simulink model "BirdHeadModel2"  (R2023a)
settings: Solver=VariableStepAuto  StartTime=0.0  StopTime=30  RelTol=1e-3
values from neighbouring files (symbols this model uses):
  dt = 0.002    [LaunchBirdHeadModel2.m]    (also in LaunchBirdHeadModelControlled.m; LaunchBirdHeadModelControlled_MovementControl.m; PlotMovementControl.m; PlotPositionControl.m)
  g = 9.81    [LaunchBirdHeadModel2.m]    (also in LaunchBirdHeadModelControlled.m; LaunchBirdHeadModelControlled_MovementControl.m; PlotMovementControl.m; PlotPositionControl.m)
  I_by = 0.00001    (= 1e-05)    [LaunchBirdHeadModel2.m]    (also in LaunchBirdHeadModelControlled.m; LaunchBirdHeadModelControlled_MovementControl.m; PlotMovementControl.m; PlotPositionControl.m)
  I_hy = 0.00001    (= 1e-05)    [LaunchBirdHeadModel2.m]    (also in LaunchBirdHeadModelControlled.m; LaunchBirdHeadModelControlled_MovementControl.m; PlotMovementControl.m; PlotPositionControl.m)
  Kp = [20  0; 0  20]    [CondIni-1010Kp201Kv101.mat]    (also in Kp101Kv51.mat = [20  0; 0  1]; Kp11Kv051.mat = [1  0; 0  1]; Kp11Kv11.mat = [1  0; 0  1]; Kp11Kv21.mat = [1  0; 0  1])
  Kv = [10  0; 0  10]    [CondIni-1010Kp201Kv101.mat]    (also in Kp101Kv51.mat = [5  0; 0  1]; Kp11Kv051.mat = [0.5  0; 0  1]; Kp11Kv11.mat = [1  0; 0  1]; Kp11Kv21.mat = [2  0; 0  1])
  l_b = 0.05    [LaunchBirdHeadModel2.m]    (also in LaunchBirdHeadModelControlled.m; LaunchBirdHeadModelControlled_MovementControl.m; PlotMovementControl.m; PlotPositionControl.m)
  l_h = 0.04    [LaunchBirdHeadModel2.m]    (also in LaunchBirdHeadModelControlled.m; LaunchBirdHeadModelControlled_MovementControl.m; PlotMovementControl.m; PlotPositionControl.m)
  m_h = 0.005    [LaunchBirdHeadModel2.m]    (also in LaunchBirdHeadModelControlled.m; LaunchBirdHeadModelControlled_MovementControl.m; PlotMovementControl.m; PlotPositionControl.m)
settings Model: Creator=coquet  LastModifiedBy=coquet

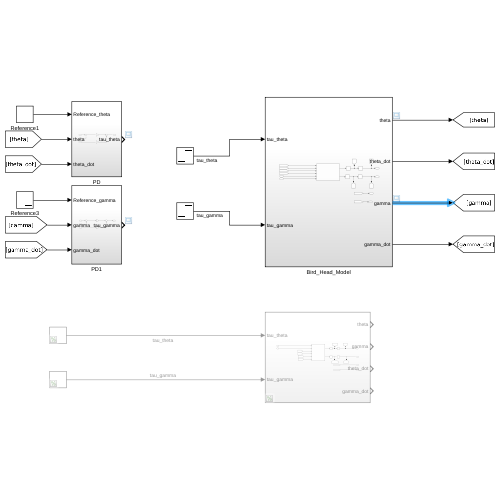
[thumbnail: Simulink's stored preview of the top-level diagram]
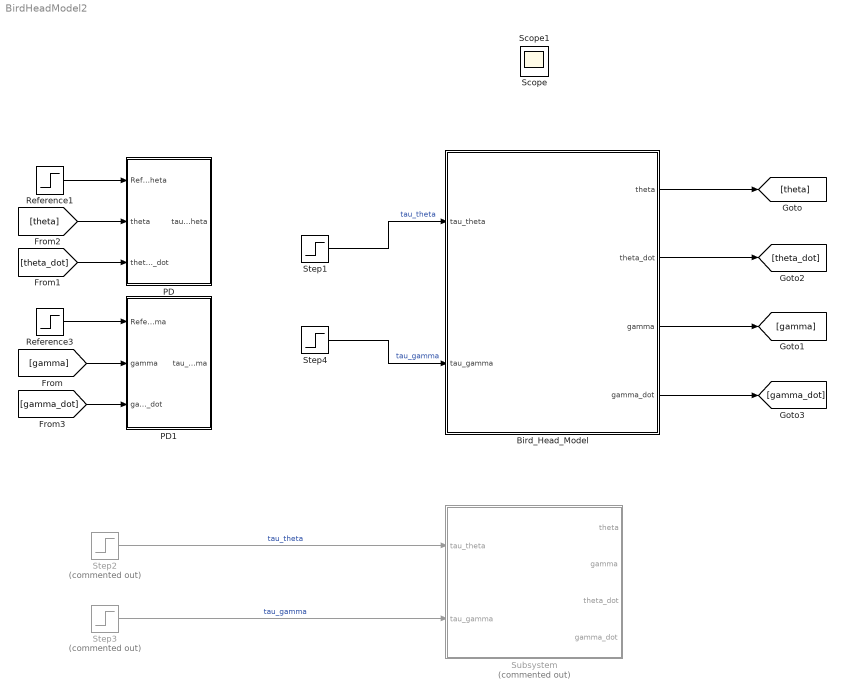
== system BirdHeadModel2 ==
  Bird_Head_Model : Subsystem
  PD : Subsystem
  PD1 : Subsystem
  Reference1 : Step  Time=5  After=8*pi/60  SampleTime=0
  Reference3 : Step  Time=5  After=-8*pi/60  SampleTime=0
  Step1 : Step  After=0  SampleTime=dt
  Step2 : Step  Commented=on  After=0.001  SampleTime=0
  Step3 : Step  Commented=on  After=0.001  SampleTime=0
  Step4 : Step  After=0  SampleTime=dt
  Subsystem : Subsystem  Commented=on
  Scope : Scope
  Scope1 : Scope
  wires:
  [gamma] -> PD1/2(gamma)
  [theta] -> PD/2(theta)
  Reference1/1 -> PD/1(Reference_theta)
  Reference3/1 -> PD1/1(Reference_gamma)
  Bird_Head_Model/1(theta) -> [theta]
  Bird_Head_Model/3(gamma) -> [gamma]
  [theta_dot] -> PD/3(theta_dot)
  Bird_Head_Model/2(theta_dot) -> [theta_dot]
  Bird_Head_Model/4(gamma_dot) -> [gamma_dot]
  [gamma_dot] -> PD1/3(gamma_dot)
  Step3/1 -> Subsystem/2(tau_gamma)  "tau_gamma"
  Step2/1 -> Subsystem/1(tau_theta)  "tau_theta"
  Step1/1 -> Bird_Head_Model/1(tau_theta)  "tau_theta"
  Step4/1 -> Bird_Head_Model/2(tau_gamma)  "tau_gamma"

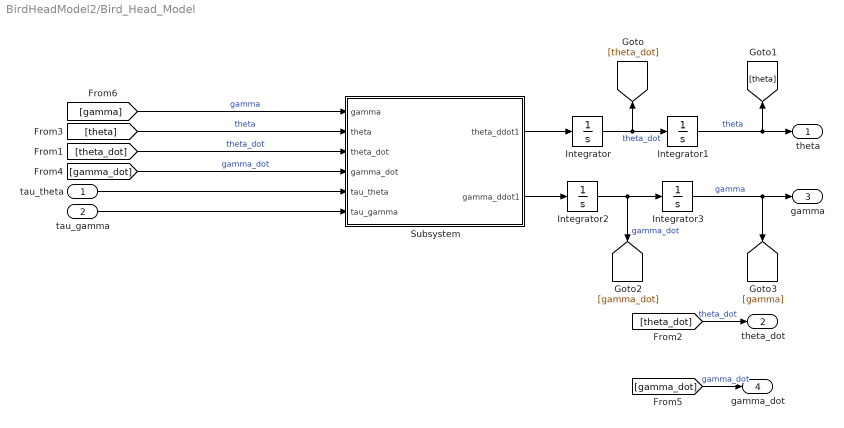
== system BirdHeadModel2/Bird_Head_Model ==
  tau_theta : Inport
  tau_gamma : Inport  Port=2
  Integrator : Integrator  ContinuousStateAttributes='theta_dot'
  Integrator1 : Integrator  UpperSaturationLimit=2*pi/9  LowerSaturationLimit=-pi/3  WrapState=on  ContinuousStateAttributes='theta'
  Integrator2 : Integrator  ContinuousStateAttributes='gamma_dot'
  Integrator3 : Integrator  UpperSaturationLimit=2*pi/9  LowerSaturationLimit=-pi/3  WrapState=on  ContinuousStateAttributes='gamma'
  Subsystem : Subsystem
  theta : Outport
  theta_dot : Outport  Port=2
  gamma : Outport  Port=3
  gamma_dot : Outport  Port=4
  wires:
  Subsystem/1(theta_ddot1) -> Integrator/1
  [theta] -> Subsystem/2(theta)  "theta"
  [gamma_dot] -> Subsystem/4(gamma_dot)  "gamma_dot"
  Subsystem/2(gamma_ddot1) -> Integrator2/1
  [theta_dot] -> Subsystem/3(theta_dot)  "theta_dot"
  [gamma] -> Subsystem/1(gamma)  "gamma"
  Integrator1/1 -> theta/1, [theta]  "theta"
  Integrator2/1 -> [gamma_dot], Integrator3/1  "gamma_dot"
  Integrator/1 -> Integrator1/1, [theta_dot]  "theta_dot"
  tau_gamma/1 -> Subsystem/6(tau_gamma)
  Integrator3/1 -> gamma/1, [gamma]  "gamma"
  tau_theta/1 -> Subsystem/5(tau_theta)
  [theta_dot] -> theta_dot/1  "theta_dot"
  [gamma_dot] -> gamma_dot/1  "gamma_dot"

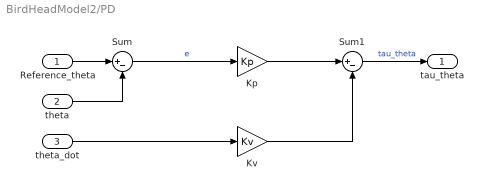
== system BirdHeadModel2/PD ==
  Reference_theta : Inport
  theta : Inport  Port=2
  theta_dot : Inport  Port=3
  Kp : Gain  Gain=Kp
  Kv : Gain  Gain=Kv
  Sum : Sum  Inputs=|+-
  Sum1 : Sum  Inputs=|+-
  tau_theta : Outport
  wires:
  Sum/1 -> Kp/1  "e"
  Kv/1 -> Sum1/2
  theta/1 -> Sum/2
  Reference_theta/1 -> Sum/1
  Kp/1 -> Sum1/1
  Sum1/1 -> tau_theta/1  "tau_theta"
  theta_dot/1 -> Kv/1

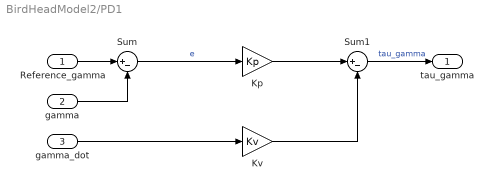
== system BirdHeadModel2/PD1 ==
  Reference_gamma : Inport
  gamma : Inport  Port=2
  gamma_dot : Inport  Port=3
  Kp : Gain  Gain=Kp
  Kv : Gain  Gain=Kv
  Sum : Sum  Inputs=|+-
  Sum1 : Sum  Inputs=|+-
  tau_gamma : Outport
  wires:
  Sum/1 -> Kp/1  "e"
  Kv/1 -> Sum1/2
  gamma/1 -> Sum/2
  Reference_gamma/1 -> Sum/1
  Kp/1 -> Sum1/1
  Sum1/1 -> tau_gamma/1  "tau_gamma"
  gamma_dot/1 -> Kv/1

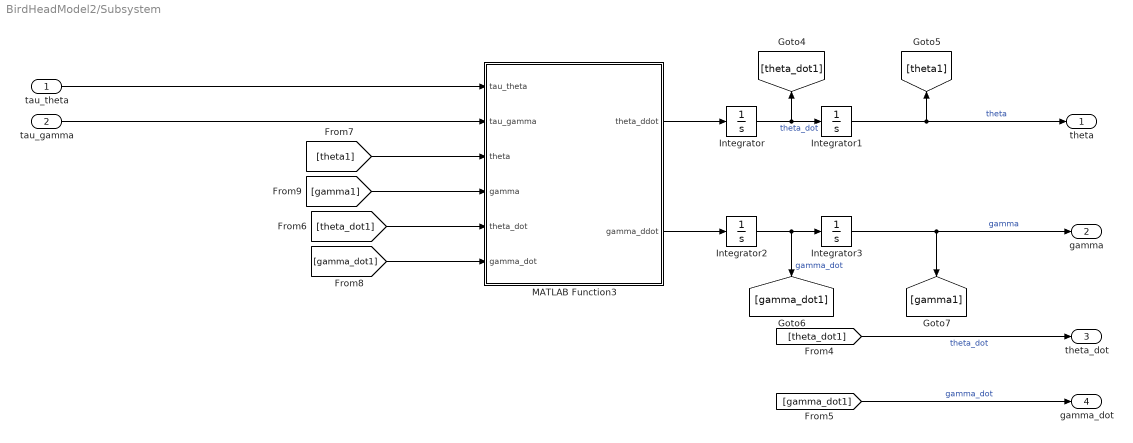
== system BirdHeadModel2/Subsystem ==
  tau_theta : Inport
  tau_gamma : Inport  Port=2
  Integrator : Integrator  ContinuousStateAttributes='theta_dot'
  Integrator1 : Integrator  UpperSaturationLimit=2*pi/9  LowerSaturationLimit=-pi/3  ContinuousStateAttributes='theta'
  Integrator2 : Integrator  ContinuousStateAttributes='gamma_dot'
  Integrator3 : Integrator  UpperSaturationLimit=2*pi/9  LowerSaturationLimit=-pi/3  ContinuousStateAttributes='gamma'
  MATLAB Function3 : MATLAB Function  TreatAsAtomicUnit=on
  theta : Outport
  gamma : Outport  Port=2
  theta_dot : Outport  Port=3
  gamma_dot : Outport  Port=4
  wires:
  [gamma1] -> MATLAB Function3/4(gamma)
  Integrator1/1 -> theta/1, [theta1]  "theta"
  [theta1] -> MATLAB Function3/3(theta)
  tau_theta/1 -> MATLAB Function3/1(tau_theta)
  [theta_dot1] -> MATLAB Function3/5(theta_dot)
  MATLAB Function3/1(theta_ddot) -> Integrator/1
  [gamma_dot1] -> MATLAB Function3/6(gamma_dot)
  [theta_dot1] -> theta_dot/1  "theta_dot"
  MATLAB Function3/2(gamma_ddot) -> Integrator2/1
  Integrator3/1 -> gamma/1, [gamma1]  "gamma"
  tau_gamma/1 -> MATLAB Function3/2(tau_gamma)
  Integrator2/1 -> [gamma_dot1], Integrator3/1  "gamma_dot"
  [gamma_dot1] -> gamma_dot/1  "gamma_dot"
  Integrator/1 -> Integrator1/1, [theta_dot1]  "theta_dot"

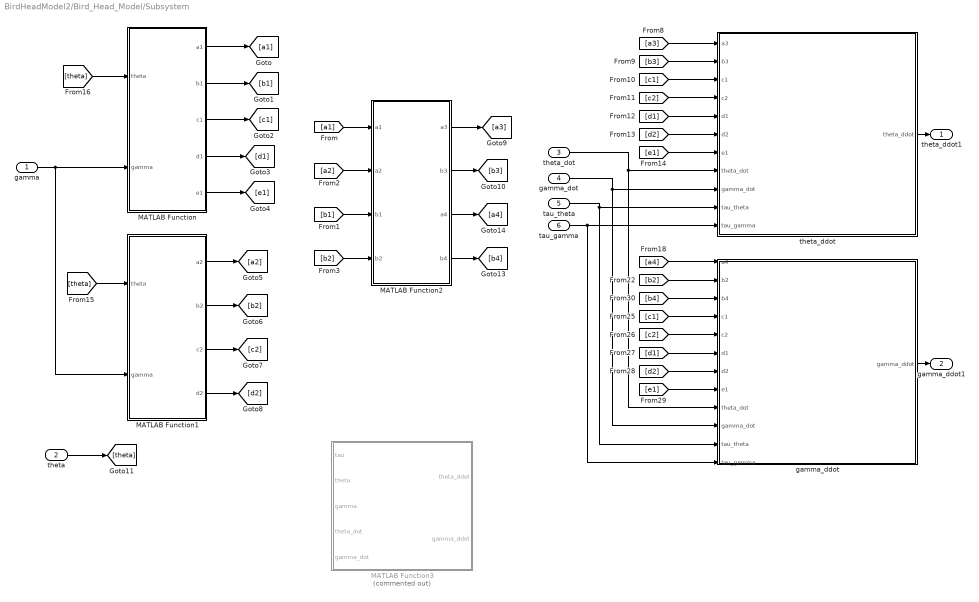
== system BirdHeadModel2/Bird_Head_Model/Subsystem ==
  gamma : Inport
  theta : Inport  Port=2
  theta_dot : Inport  Port=3
  gamma_dot : Inport  Port=4
  tau_theta : Inport  Port=5
  tau_gamma : Inport  Port=6
  MATLAB Function : MATLAB Function  TreatAsAtomicUnit=on
  MATLAB Function1 : MATLAB Function  TreatAsAtomicUnit=on
  MATLAB Function2 : MATLAB Function  TreatAsAtomicUnit=on
  MATLAB Function3 : MATLAB Function  Commented=on  TreatAsAtomicUnit=on
  gamma_ddot : MATLAB Function  TreatAsAtomicUnit=on
  theta_ddot : MATLAB Function  TreatAsAtomicUnit=on
  theta_ddot1 : Outport
  gamma_ddot1 : Outport  Port=2
  wires:
  [c2] -> gamma_ddot/5(c2)
  [e1] -> gamma_ddot/8(e1)
  [d2] -> theta_ddot/6(d2)
  theta_ddot/1(theta_ddot) -> theta_ddot1/1
  [a4] -> gamma_ddot/1(a4)
  [c2] -> theta_ddot/4(c2)
  [b2] -> gamma_ddot/2(b2)
  [d2] -> gamma_ddot/7(d2)
  tau_theta/1 -> gamma_ddot/11(tau_theta), theta_ddot/10(tau_theta)
  [e1] -> theta_ddot/7(e1)
  gamma_ddot/1(gamma_ddot) -> gamma_ddot1/1
  theta/1 -> [theta]
  tau_gamma/1 -> gamma_ddot/12(tau_gamma), theta_ddot/11(tau_gamma)
  [d1] -> theta_ddot/5(d1)
  [c1] -> gamma_ddot/4(c1)
  [b3] -> theta_ddot/2(b3)
  [c1] -> theta_ddot/3(c1)
  theta_dot/1 -> gamma_ddot/9(theta_dot), theta_ddot/8(theta_dot)
  [b4] -> gamma_ddot/3(b4)
  gamma_dot/1 -> gamma_ddot/10(gamma_dot), theta_ddot/9(gamma_dot)
  [d1] -> gamma_ddot/6(d1)
  [a3] -> theta_ddot/1(a3)
  MATLAB Function/1(a1) -> [a1]
  MATLAB Function/2(b1) -> [b1]
  MATLAB Function/3(c1) -> [c1]
  MATLAB Function/4(d1) -> [d1]
  MATLAB Function/5(e1) -> [e1]
  gamma/1 -> MATLAB Function/2(gamma), MATLAB Function1/2(gamma)
  [theta] -> MATLAB Function/1(theta)
  MATLAB Function1/1(a2) -> [a2]
  MATLAB Function1/2(b2) -> [b2]
  MATLAB Function1/3(c2) -> [c2]
  MATLAB Function1/4(d2) -> [d2]
  [theta] -> MATLAB Function1/1(theta)
  [a1] -> MATLAB Function2/1(a1)
  [a2] -> MATLAB Function2/2(a2)
  [b1] -> MATLAB Function2/3(b1)
  [b2] -> MATLAB Function2/4(b2)
  MATLAB Function2/1(a3) -> [a3]
  MATLAB Function2/2(b3) -> [b3]
  MATLAB Function2/3(a4) -> [a4]
  MATLAB Function2/4(b4) -> [b4]

== matlab function BirdHeadModel2/Bird_Head_Model/Subsystem/MATLAB Function1 ==
  data: theta input; a2 output; gamma input; b2 output; c2 output; d2 output; m_h parameter; l_b parameter; l_h parameter; I_hy parameter; I_by parameter; g parameter
function [a2, b2, c2, d2] = coefs2(theta, gamma, m_h, l_b, l_h, I_hy, I_by, g)
a2 = I_hy+l_h^2*m_h+l_b*l_h*m_h*cos(gamma);
b2 = I_hy + l_h^2*m_h;
c2 = l_b*l_h*m_h*sin(gamma);
d2 = -l_h*m_h*cos(gamma+theta);

== matlab function BirdHeadModel2/Bird_Head_Model/Subsystem/MATLAB Function2 ==
  data: a1 input; a2 input; b1 input; a3 output; b3 output; a4 output; b4 output; b2 input
function [a3, b3, a4, b4] = coefs3(a1, a2, b1, b2)

a3 = (b1/(a2*b1-a1*b2));
b3 = (b2/(a2*b1-a1*b2));
a4 = a3*a2/b2;
b4 = b3*a2/b2;

== matlab function BirdHeadModel2/Bird_Head_Model/Subsystem/gamma_ddot ==
  data: a4 input; gamma_ddot output; b2 input; b4 input; c1 input; c2 input; d1 input; d2 input; e1 input; theta_dot input; gamma_dot input; tau_theta input; tau_gamma input
function gamma_ddot = fcn(a4,b2,b4, c1,c2,d1,d2,e1,theta_dot, gamma_dot,tau_theta, tau_gamma)
I_hy = 0.0001;
I_by = 0.0001;
l_h = 0.040;
l_b = 0.050;
m_h = 0.0049;
g = 9.8;
gamma_ddot = tau_gamma * (1/b2 - a4) + (a4*c2-c2/b2)*theta_dot^2 + (a4*d2-b4*e1-d2/b2)*g + b4*tau_theta -b4*c1*gamma_dot^2 - b4*d1*theta_dot*gamma_dot;

== matlab function BirdHeadModel2/Bird_Head_Model/Subsystem/MATLAB Function3 ==
  data: tau input; theta_ddot output; theta input; gamma input; theta_dot input; gamma_dot input; gamma_ddot output; I_hy parameter; m_h parameter; l_b parameter; l_h parameter; I_by parameter
function [theta_ddot, gamma_ddot] = fcn(tau,theta,gamma,theta_dot,gamma_dot, I_hy, m_h, l_b, l_h, I_by)

m11 = I_hy+I_by+(l_b^2+l_h^2)*m_h+ 2*l_b*l_h*m_h*cos(gamma);
m12 = I_hy+l_h^2*m_h*sin(2*gamma)+l_b*l_h*m_h*sin(gamma);
m21 = I_hy+l_h^2*m_h*sin(2*gamma) + l_b*l_h*m_h*sin(gamma);
m22 = I_hy + l_h^2*m_h;

M=[m11 m12;
   m21 m22];


c11 = -2*l_b*l_h *m_h*sin(gamma)*gamma_dot;
c12 = (2*l_h^2*m_h*cos(2*gamma) + l_b*l_h*m_h*cos(gamma))*gamma_dot;
c21 = l_b*l_h*m_h*sin(gamma)*theta_dot;
c22 = 0;

C=[c11 c12; 
   c21 c22];

g1 = -l_h*m_h*sin(gamma - theta)+l_b*m_h*sin(theta);
g2 = l_h*m_h*cos(gamma + theta);

G=[g1;g2];

qddot=M\(tau-C*[theta_dot;gamma_dot]-G);

theta_ddot=qddot(1);
gamma_ddot=qddot(2);

== matlab function BirdHeadModel2/Subsystem/MATLAB Function3 ==
  data: tau_theta input; tau_gamma input; theta_ddot output; theta input; gamma input; theta_dot input; gamma_dot input; gamma_ddot output; I_hy parameter; m_h parameter; l_b parameter; l_h parameter; I_by parameter
function [theta_ddot, gamma_ddot] = fcn(tau_theta, tau_gamma,theta,gamma,theta_dot,gamma_dot, I_hy, m_h, l_b, l_h, I_by)

tau = [tau_theta, tau_gamma];

m11 = I_hy+I_by+(l_b^2+l_h^2)*m_h+ 2*l_b*l_h*m_h*cos(gamma);
m12 = I_hy+l_h^2*m_h*sin(2*gamma)+l_b*l_h*m_h*sin(gamma);
m21 = I_hy+l_h^2*m_h*sin(2*gamma) + l_b*l_h*m_h*sin(gamma);
m22 = I_hy + l_h^2*m_h;

M=[m11 m12;
   m21 m22];


c11 = -2*l_b*l_h *m_h*sin(gamma)*gamma_dot;
c12 = (2*l_h^2*m_h*cos(2*gamma) + l_b*l_h*m_h*cos(gamma))*gamma_dot;
c21 = l_b*l_h*m_h*sin(gamma)*theta_dot;
c22 = 0;

C=[c11 c12; 
   c21 c22];

g1 = l_b*m_h*sin(theta)-l_h*m_h*sin(gamma - theta);
g2 = l_h*m_h*cos(gamma + theta);

G=[g1;g2];

qddot=M\(tau-C*[theta_dot;gamma_dot]-G);

theta_ddot=qddot(1);
gamma_ddot=qddot(2);

== matlab function BirdHeadModel2/Bird_Head_Model/Subsystem/theta_ddot ==
  data: a3 input; theta_ddot output; b3 input; c1 input; c2 input; d1 input; d2 input; e1 input; theta_dot input; gamma_dot input; tau_theta input; tau_gamma input
function theta_ddot = fcn(a3,b3,c1,c2,d1,d2,e1,theta_dot, gamma_dot,tau_theta, tau_gamma)
I_by=0.00003;
I_hy=0.00005;
l_b=0.1;
l_h=0.05;
m_b=0.51;
m_h=0.005;
g = 9.8;
theta_ddot = a3*tau_gamma - a3*c2*theta_dot^2 - a3*d2*g -b3*tau_theta + b3*c1*gamma_dot^2 + b3*d1*theta_dot*gamma_dot + b3*e1*g ;

== matlab function BirdHeadModel2/Bird_Head_Model/Subsystem/MATLAB Function ==
  data: theta input; a1 output; gamma input; b1 output; c1 output; d1 output; e1 output; m_h parameter; l_b parameter; l_h parameter; I_hy parameter; I_by parameter; g parameter
function [a1, b1, c1, d1, e1] = coefs1(theta, gamma, m_h,l_b,  l_h, I_hy, I_by, g)
a1 = I_hy+I_by+(l_b^2+l_h^2)*m_h+2*l_b*l_h*m_h*cos(gamma);
b1 = I_hy+l_h^2*m_h+l_b*l_h*m_h*cos(gamma);
c1 = -l_b*l_h*m_h*sin(gamma);
d1 = -2*l_b*l_h*m_h*sin(gamma);
e1 = -m_h*cos(gamma)*(l_b+l_h*cos(gamma))+l_h*m_h*sin(gamma)*sin(theta);
